simulink model "RoboBoatVU_2014_Athena"  (R2014a)
settings: Solver=FixedStepDiscrete  StartTime=0.0  StopTime=inf  FixedStep=.1  RelTol=1e-3
undefined symbols (not defined in the file): Com1, Com2, Com3, Com4, DiscIntNeverNeededParam, RGB24, standard, strel
libraries: visiontextngfix x25, dspmtrx3 x22, simulink x19, xpcseriallib x12, slrtlib x7, speedgoatlib_IO102 x6, dspstat3 x5, visionstatistics x3, dspindex x2, xpcvideousblib x2, xpcvideoutillib x2, visionmorphops x1
(part 3 of 4)

== system RoboBoatVU_2014_Athena/Main FSM/Return to Start/GPS: Center/Approach ==
  Sensors : Inport
  RGB image : Inport  Port=2
  Enable : EnablePort
  Annotate Task : visiontextngfix/Insert Text  inputType=Obsolete  theText='GPS - Center: Approach - Distance: %f'  getTextLocFrom=Specify via dialog  textLoc=[10 70]  getTextColorFrom=Specify via dialog  textColor=[255 0 0]  getTextIntensityFrom=Specify via dialog  textIntensity=0  getTextOpacityFrom=Specify via dialog  textOpacity=1.0  dummyVar2=0  dummyVar3=0  dummyVar4=0  imagePorts=One multidimensional signal  isInputTransposed=off  fontFace=LucidaSansRegular  dummyVar1=0  blockFontSize=12  antiAliased=on
  Annotate Task2 : visiontextngfix/Insert Text  inputType=Obsolete  theText='Return to Start'  getTextLocFrom=Specify via dialog  textLoc=[1 1]  getTextColorFrom=Specify via dialog  textColor=[0 0 0]  getTextIntensityFrom=Specify via dialog  textIntensity=0  getTextOpacityFrom=Specify via dialog  textOpacity=1.0  dummyVar2=0  dummyVar3=0  dummyVar4=0  imagePorts=One multidimensional signal  isInputTransposed=off  fontFace=LucidaSansRegular  dummyVar1=0  blockFontSize=12  antiAliased=on
  Bus Selector : BusSelector  OutputSignals=Serial In.GPS.latitude,Serial In.GPS.longitude
  Data Store Read : DataStoreRead  DataStoreName=colorGPS  SampleTime=0.1
  Desired Heading and Distance : MATLAB Function  TreatAsAtomicUnit=on
  Output Heirarchy : Subsystem
  Read1 : DataStoreRead  DataStoreName=GPSapproachDist  SampleTime=0.1
  Within Range : MATLAB Function  TreatAsAtomicUnit=on
  Outputs : Outport
  wires:
  Sensors/1 -> Output Heirarchy/4(Sensors), Bus Selector/1  "Sensors"
  Data Store Read/1 -> Desired Heading and Distance/1(DesiredGPS)
  Bus Selector/1 -> Desired Heading and Distance/2(GPSLat)  "<latitude>"
  Bus Selector/2 -> Desired Heading and Distance/3(GPSLong)  "<longitude>"
  Desired Heading and Distance/2(DesiredHeading) -> Output Heirarchy/2(Desired Heading)
  Annotate Task/1 -> Output Heirarchy/3(Annotated Image)
  RGB image/1 -> Annotate Task2/1
  Desired Heading and Distance/1(Distance) -> Annotate Task/2, Within Range/2(Distance)
  Read1/1 -> Within Range/1(GPSApproachDist)
  Within Range/1(Finished) -> Output Heirarchy/1(Finished)  "Task Finished"
  Output Heirarchy/1(Outputs) -> Outputs/1
  Annotate Task2/1 -> Annotate Task/1

== system RoboBoatVU_2014_Athena/Main FSM/Return to Start/GPS: Center/Orient ==
  Sensors : Inport
  RGB image : Inport  Port=2
  Enable : EnablePort
  Annotate Task : visiontextngfix/Insert Text  inputType=Obsolete  theText='GPS - Center: Orient %f'  getTextLocFrom=Specify via dialog  textLoc=[10 70]  getTextColorFrom=Specify via dialog  textColor=[255 0 0]  getTextIntensityFrom=Specify via dialog  textIntensity=0  getTextOpacityFrom=Specify via dialog  textOpacity=1.0  dummyVar2=0  dummyVar3=0  dummyVar4=0  imagePorts=One multidimensional signal  isInputTransposed=off  fontFace=LucidaSansRegular  dummyVar1=0  blockFontSize=12  antiAliased=on
  Annotate Task1 : visiontextngfix/Insert Text  inputType=Obsolete  theText='Current Heading %f'  getTextLocFrom=Specify via dialog  textLoc=[10 40]  getTextColorFrom=Specify via dialog  textColor=[255 0 0]  getTextIntensityFrom=Specify via dialog  textIntensity=0  getTextOpacityFrom=Specify via dialog  textOpacity=1.0  dummyVar2=0  dummyVar3=0  dummyVar4=0  imagePorts=One multidimensional signal  isInputTransposed=off  fontFace=LucidaSansRegular  dummyVar1=0  blockFontSize=12  antiAliased=on
  Annotate Task2 : visiontextngfix/Insert Text  inputType=Obsolete  theText='Return to Start'  getTextLocFrom=Specify via dialog  textLoc=[1 1]  getTextColorFrom=Specify via dialog  textColor=[0 0 0]  getTextIntensityFrom=Specify via dialog  textIntensity=0  getTextOpacityFrom=Specify via dialog  textOpacity=1.0  dummyVar2=0  dummyVar3=0  dummyVar4=0  imagePorts=One multidimensional signal  isInputTransposed=off  fontFace=LucidaSansRegular  dummyVar1=0  blockFontSize=12  antiAliased=on
  Bus Selector : BusSelector  OutputSignals=Serial In.GPS.latitude,Serial In.GPS.longitude,Serial In.Compass.Heading
  Data Store Read : DataStoreRead  DataStoreName=colorGPS  SampleTime=0.1
  Desired Heading : MATLAB Function  TreatAsAtomicUnit=on
  Output Heirarchy1 : Subsystem
  Within Range : MATLAB Function  TreatAsAtomicUnit=on
  Outputs : Outport
  Finished : Outport  Port=2
  wires:
  Sensors/1 -> Output Heirarchy1/3(Sensors), Bus Selector/1  "Sensors"
  Data Store Read/1 -> Desired Heading/1(DesiredGPS)
  Bus Selector/1 -> Desired Heading/2(GPSLat)  "<latitude>"
  Bus Selector/2 -> Desired Heading/3(GPSLong)  "<longitude>"
  Desired Heading/1(DesiredHeading) -> Output Heirarchy1/2(Desired Heading), Annotate Task/2, Within Range/1(DesiredHeading)
  Bus Selector/3 -> Annotate Task1/2, Within Range/2(Compass)  "<Heading>"
  Within Range/1(Finished) -> Finished/1
  RGB image/1 -> Annotate Task2/1
  Output Heirarchy1/1(Outputs) -> Outputs/1
  Annotate Task/1 -> Annotate Task1/1
  Annotate Task1/1 -> Output Heirarchy1/1(Annotated Image)
  Annotate Task2/1 -> Annotate Task/1

== system RoboBoatVU_2014_Athena/Main FSM/Return to Start/GPS: Center/Output Reassign ==
  Outputs in : Inport
  Bus Selector : BusSelector  OutputSignals=Task Finished,Output Signals
  Outputs : Outport
  Finished : Outport  Port=2
  wires:
  Outputs in/1 -> Bus Selector/1
  Bus Selector/1 -> Finished/1  "<Task Finished>"
  Bus Selector/2 -> Outputs/1  "<Output Signals>"

== system RoboBoatVU_2014_Athena/Main FSM/Start Speed Gate/Start Speed Gate - Color/Buoy Decisions ==
  Sensors : Inport
  RGB image : Inport  Port=2
  Red + Green : Inport  Port=3
  Timer : Inport  Port=4
  Annotate Image : Subsystem
  Bus Selector : BusSelector  OutputSignals=Serial In.Compass.Heading
  Bus Selector1 : BusSelector  OutputSignals=Red BBox,Green BBox,Red Centroid,Green Centroid
  Nav Logic : MATLAB Function  TreatAsAtomicUnit=on
  Read : DataStoreRead  DataStoreName=Course
  Annotated Image : Outport
  RPM : Outport  Port=2
  Desired Heading : Outport  Port=3
  wires:
  RGB image/1 -> Annotate Image/1(RGB image)
  Red + Green/1 -> Bus Selector1/1
  Annotate Image/1(Annotated Image) -> Annotated Image/1
  Bus Selector1/1 -> Annotate Image/2(Red BBox), Nav Logic/2(RedBBox)  "<Red BBox>"
  Bus Selector1/2 -> Annotate Image/3(Green BBox), Nav Logic/3(GreenBBox)  "<Green BBox>"
  Bus Selector1/3 -> Nav Logic/4(RedCentroid)  "<Red Centroid>"
  Bus Selector1/4 -> Nav Logic/5(GreenCentroid)  "<Green Centroid>"
  Bus Selector/1 -> Nav Logic/1(Compass)  "<Heading>"
  Sensors/1 -> Bus Selector/1
  Nav Logic/1(RedDist) -> Annotate Image/4(Red Dist)
  Nav Logic/2(GreenDist) -> Annotate Image/5(Green Dist)
  Nav Logic/3(RPM) -> RPM/1
  Nav Logic/4(DesiredHeading) -> Desired Heading/1
  Read/1 -> Nav Logic/6(Course)
  Timer/1 -> Nav Logic/7(Timer)

== system RoboBoatVU_2014_Athena/Main FSM/Start Speed Gate/Start Speed Gate - Color/Output Heirarchy ==
  Sensors : Inport
  Annotated Image : Inport  Port=2
  RPM : Inport  Port=3
  Desired Heading : Inport  Port=4
  Finished : Inport  Port=5
  Bus Creator : BusCreator  Inputs=3
  Bus Creator1 : BusCreator  Inputs=2
  Bus Creator2 : BusCreator  Inputs=3
  Bus Creator3 : BusCreator  Inputs=2
  Bus Creator4 : BusCreator  Inputs=2
  Due Sample Start : Constant  Value=0
  Ready to Read : Constant  Value=0
  Uno Power : Constant  Value=0
  Outputs : Outport
  wires:
  RPM/1 -> Bus Creator/1  "RPM"
  Bus Creator/1 -> Bus Creator1/1  "Control Signals"
  Bus Creator2/1 -> Bus Creator/3  "Arduino Signals"
  Uno Power/1 -> Bus Creator2/2  "Uno Power"
  Desired Heading/1 -> Bus Creator/2  "Desired Heading"
  Bus Creator1/1 -> Bus Creator4/1  "Outputs"
  Annotated Image/1 -> Bus Creator1/2  "Annotated Image"
  Sensors/1 -> Bus Creator4/2  "Sensors"
  Bus Creator4/1 -> Bus Creator3/1  "Output Signals"
  Ready to Read/1 -> Bus Creator2/1  "Ready to Read"
  Due Sample Start/1 -> Bus Creator2/3  "Due Sample Start"
  Finished/1 -> Bus Creator3/2  "Task Finished"
  Bus Creator3/1 -> Outputs/1

== system RoboBoatVU_2014_Athena/Main FSM/Start Speed Gate/Start Speed Gate - Color/Start Speed Gate Detection ==
  RGB : Inport
  Bus Creator : BusCreator
  Green Detection : Subsystem
  Red Detection : Subsystem
  S-Function : S-Function  FunctionName=rgbtohsv_int_sfun  EnableBusSupport=off
  Red + Green : Outport
  wires:
  RGB/1 -> S-Function/1
  S-Function/1 -> Green Detection/1(HSV), Red Detection/1(HSV)
  Red Detection/1(Red Centroid) -> Bus Creator/1  "Red Centroid"
  Red Detection/2(Red BBox) -> Bus Creator/2  "Red BBox"
  Green Detection/1(Green Centroid) -> Bus Creator/3  "Green Centroid"
  Green Detection/2(Green BBox) -> Bus Creator/4  "Green BBox"
  Bus Creator/1 -> Red + Green/1

== matlab function RoboBoatVU_2014_Athena/Parameters/GPS Points/GPS Selector ==
  data: course input; ssGate output; rtnIn input; ssGateA input; colorA input; obstNavStartA input; obstNavEndA input; acouLocA input; dockA input; ssGateB input; colorB input; obstNavStartB input; obstNavEndB input; acouLocB input; dockB input; ssGateT input; colorT input; obstNavStartT input; obstNavEndT input; acouLocT input; dockT input; color output; obstNavStart output; obstNavEnd output; acouLoc output; dock output; rtnOut output
function [ssGate,color,obstNavStart,obstNavEnd,acouLoc,dock,rtnOut] = ...
    GPSselector(course,rtnIn,...
    ssGateA,colorA,obstNavStartA,obstNavEndA,acouLocA,dockA,...
    ssGateB,colorB,obstNavStartB,obstNavEndB,acouLocB,dockB,...
    ssGateT,colorT,obstNavStartT,obstNavEndT,acouLocT,dockT)

%Written by: Anderson Lebbad on July 18, 2013
%Last Edited: Edward Zhu on June
%   Data type mismatch addressed
%   Character conversion redundant

%Selects GPS Points to use based on input Course

%Check value of CourseStr and pass inputs accordingly

switch course
    case uint8('A')
        ssGate = ssGateA;
        color = colorA;
        obstNavStart = obstNavStartA;
        obstNavEnd = obstNavEndA;
        acouLoc = acouLocA;
        dock = dockA;
        rtnOut = rtnIn;
        
    case uint8('B')
        ssGate = ssGateB;
        color = colorB;
        obstNavStart = obstNavStartB;
        obstNavEnd = obstNavEndB;
        acouLoc = acouLocB;
        dock = dockB;
        rtnOut = rtnIn;
        
    otherwise
        ssGate = ssGateT;
        color = colorT;
        obstNavStart = obstNavStartT;
        obstNavEnd = obstNavEndT;
        acouLoc = acouLocT;
        dock = dockT;
        rtnOut = rtnIn;
end

== matlab function RoboBoatVU_2014_Athena/Parameters/Task Selector/Message Composer3 ==
  data: taskStrInit input; taskStrAdj output
function taskStrAdj = composeMessage(taskStrInit)
%Written by Anderson Lebbad on August 9, 2013
%Last Edited: Edward Zhu on June 2, 2014

%This function adjusts the length of a vector to a set value by filling
%the remaining space with 0's. This is necessary for data store objects
%that have a fixed size for the memory allocation, but a variable length
%input.

%Length of message packet
strLength = 8;

%Size of text in message
taskStrLength = size(taskStrInit,1);

%Pad end of text with zeros
taskStrAdj = [taskStrInit' zeros(1,strLength-taskStrLength)];

== matlab function RoboBoatVU_2014_Athena/Parameters/Task Selector/Message Composer6 ==
  data: taskStrInit input; taskStrAdj output
function taskStrAdj = composeMessage(taskStrInit)
%Written by Anderson Lebbad on August 9, 2013
%Last Edited: Edward Zhu on June 2, 2014

%This function adjusts the length of a vector to a set value by filling
%the remaining space with 0's. This is necessary for data store objects
%that have a fixed size for the memory allocation, but a variable length
%input.

%Length of message packet
strLength = 8;

%Size of text in message
taskStrLength = size(taskStrInit,1);

%Pad end of text with zeros
taskStrAdj = [taskStrInit' zeros(1,strLength-taskStrLength)];

== system RoboBoatVU_2014_Athena/Main FSM/Start Speed Gate/Start Speed Gate - LIDAR/Output Heirarchy ==
  Sensors : Inport
  Annotated Image : Inport  Port=2
  RPM : Inport  Port=3
  Desired Heading : Inport  Port=4
  Finished : Inport  Port=5
  Bus Creator : BusCreator  Inputs=3
  Bus Creator1 : BusCreator  Inputs=2
  Bus Creator2 : BusCreator  Inputs=3
  Bus Creator3 : BusCreator  Inputs=2
  Bus Creator4 : BusCreator  Inputs=2
  Due Sample Start : Constant  Value=0
  Ready to Read : Constant  Value=0
  Uno Power : Constant  Value=0
  Outputs : Outport
  wires:
  RPM/1 -> Bus Creator/1  "RPM"
  Bus Creator/1 -> Bus Creator1/1  "Control Signals"
  Bus Creator2/1 -> Bus Creator/3  "Arduino Signals"
  Uno Power/1 -> Bus Creator2/2  "Uno Power"
  Desired Heading/1 -> Bus Creator/2  "Desired Heading"
  Bus Creator1/1 -> Bus Creator4/1  "Outputs"
  Annotated Image/1 -> Bus Creator1/2  "Annotated Image"
  Sensors/1 -> Bus Creator4/2  "Sensors"
  Bus Creator4/1 -> Bus Creator3/1  "Output Signals"
  Ready to Read/1 -> Bus Creator2/1  "Ready to Read"
  Due Sample Start/1 -> Bus Creator2/3  "Due Sample Start"
  Finished/1 -> Bus Creator3/2  "Task Finished"
  Bus Creator3/1 -> Outputs/1

== system RoboBoatVU_2014_Athena/Sensors/Serial In/Decode Compass/Correct Heading Angle Magnetic to True North ==
  Heading Mag : Inport
  Magnetic to True North Conversion : MATLAB Function  TreatAsAtomicUnit=on
  Heading True : Outport
  wires:
  Magnetic to True North Conversion/1(HeadingT) -> Heading True/1  "Heading"
  Heading Mag/1 -> Magnetic to True North Conversion/1(HeadingM)

== system RoboBoatVU_2014_Athena/Sinks/actuators/analog output/Subsystem ==
  Compass Heading : Inport
  Control Signals : Inport  Port=2
  Bus Selector : BusSelector  OutputSignals=RPM,Desired Heading
  Heading Controller : Subsystem
  Propulsion Controller : Subsystem
  Propulsion : Outport
  Steering : Outport  Port=2
  wires:
  Control Signals/1 -> Bus Selector/1
  Bus Selector/1 -> Propulsion Controller/1(RPM)  "<RPM>"
  Propulsion Controller/1(Propulsion) -> Propulsion/1
  Bus Selector/2 -> Heading Controller/1(Heading Desired)  "<Desired Heading>"
  Compass Heading/1 -> Heading Controller/2(Compass Heading)
  Heading Controller/1(Steering) -> Steering/1

== system RoboBoatVU_2014_Athena/Main FSM/Return to Start/GPS: Center/Approach/Output Heirarchy ==
  Finished : Inport
  Desired Heading : Inport  Port=2
  Annotated Image : Inport  Port=3
  Sensors : Inport  Port=4
  Bus Creator : BusCreator  Inputs=3
  Bus Creator1 : BusCreator  Inputs=2
  Bus Creator2 : BusCreator  Inputs=3
  Bus Creator3 : BusCreator  Inputs=2
  Bus Creator4 : BusCreator  Inputs=2
  Due Sample Start : Constant  Value=0
  RPM Desired : Constant  Value=0
  Ready to Read : Constant  Value=0
  Uno Power : Constant  Value=0
  Outputs : Outport
  wires:
  RPM Desired/1 -> Bus Creator/1  "RPM"
  Bus Creator/1 -> Bus Creator1/1  "Control Signals"
  Bus Creator2/1 -> Bus Creator/3  "Arduino Signals"
  Uno Power/1 -> Bus Creator2/2  "Uno Power"
  Desired Heading/1 -> Bus Creator/2  "Desired Heading"
  Bus Creator1/1 -> Bus Creator4/1  "Outputs"
  Annotated Image/1 -> Bus Creator1/2  "Annotated Image"
  Sensors/1 -> Bus Creator4/2  "Sensors"
  Bus Creator4/1 -> Bus Creator3/1  "Output Signals"
  Ready to Read/1 -> Bus Creator2/1  "Ready to Read"
  Due Sample Start/1 -> Bus Creator2/3  "Due Sample Start"
  Bus Creator3/1 -> Outputs/1
  Finished/1 -> Bus Creator3/2  "Task Finished"

== system RoboBoatVU_2014_Athena/Main FSM/Return to Start/GPS: Center/Orient/Output Heirarchy1 ==
  Annotated Image : Inport
  Desired Heading : Inport  Port=2
  Sensors : Inport  Port=3
  Bus Creator : BusCreator  Inputs=3
  Bus Creator1 : BusCreator  Inputs=2
  Bus Creator2 : BusCreator  Inputs=3
  Bus Creator3 : BusCreator  Inputs=2
  Bus Creator4 : BusCreator  Inputs=2
  Due Sample Start : Constant  Value=0
  Finished : Constant  Value=0
  RPM Desired : Constant  Value=0
  Ready to Read : Constant  Value=0
  Uno Power : Constant  Value=0
  Outputs : Outport
  wires:
  RPM Desired/1 -> Bus Creator/1  "RPM"
  Bus Creator/1 -> Bus Creator1/1  "Control Signals"
  Bus Creator2/1 -> Bus Creator/3  "Arduino Signals"
  Uno Power/1 -> Bus Creator2/2  "Uno Power"
  Desired Heading/1 -> Bus Creator/2  "Desired Heading"
  Bus Creator1/1 -> Bus Creator4/1  "Outputs"
  Annotated Image/1 -> Bus Creator1/2  "Annotated Image"
  Sensors/1 -> Bus Creator4/2  "Sensors"
  Bus Creator4/1 -> Bus Creator3/1  "Output Signals"
  Ready to Read/1 -> Bus Creator2/1  "Ready to Read"
  Due Sample Start/1 -> Bus Creator2/3  "Due Sample Start"
  Bus Creator3/1 -> Outputs/1
  Finished/1 -> Bus Creator3/2  "Task Finished"

== system RoboBoatVU_2014_Athena/Main FSM/Start Speed Gate/Start Speed Gate - Color/Buoy Decisions/Annotate Image ==
  RGB image : Inport
  Red BBox : Inport  Port=2
  Green BBox : Inport  Port=3
  Red Dist : Inport  Port=4
  Green Dist : Inport  Port=5
  Annotate Task : visiontextngfix/Insert Text  inputType=Obsolete  theText='Buoy Navigation'  getTextLocFrom=Specify via dialog  textLoc=[10 10]  getTextColorFrom=Specify via dialog  textColor=[0 0 255]  getTextIntensityFrom=Specify via dialog  textIntensity=0  getTextOpacityFrom=Specify via dialog  textOpacity=1.0  dummyVar2=0  dummyVar3=0  dummyVar4=0  imagePorts=One multidimensional signal  isInputTransposed=off  fontFace=LucidaSansRegular  dummyVar1=0  blockFontSize=12  antiAliased=on
  Draw Green BBox : visiontextngfix/Draw Shapes  shape=Rectangles  fill=on  lineWidth=1  fillClrSource=Specify via dialog  display=User-specified value  intensity=200  color=[0 255 0]  opacity=0.6  viewport=Entire image  antialiasing=off  inType=Obsolete  imagePorts=One multidimensional signal  prodOutputMode=Binary point scaling  prodOutputWordLength=32  prodOutputFracLength=14  memoryMode=Specify word length  memoryWordLength=16  memoryFracLength=14  roundingMode=Floor  overflowMode=off
  Draw Red BBox : visiontextngfix/Draw Shapes  shape=Rectangles  fill=on  lineWidth=1  fillClrSource=Specify via dialog  display=User-specified value  intensity=200  color=[255 0 0]  opacity=0.6  viewport=Entire image  antialiasing=off  inType=Obsolete  imagePorts=One multidimensional signal  prodOutputMode=Binary point scaling  prodOutputWordLength=32  prodOutputFracLength=14  memoryMode=Specify word length  memoryWordLength=16  memoryFracLength=14  roundingMode=Floor  overflowMode=off
  Green Distance Display : visiontextngfix/Insert Text  inputType=Obsolete  theText='Green Distance: %f m'  getTextLocFrom=Specify via dialog  textLoc=[10 130]  getTextColorFrom=Specify via dialog  textColor=[0 255 0]  getTextIntensityFrom=Specify via dialog  textIntensity=0  getTextOpacityFrom=Specify via dialog  textOpacity=1.0  dummyVar2=0  dummyVar3=0  dummyVar4=0  imagePorts=One multidimensional signal  isInputTransposed=off  fontFace=LucidaSansRegular  dummyVar1=0  blockFontSize=12  antiAliased=on
  Green integer : DataTypeConversion  OutDataTypeStr=int32
  Red Distance Display : visiontextngfix/Insert Text  inputType=Obsolete  theText='Red Distance: %f m'  getTextLocFrom=Specify via dialog  textLoc=[10 70]  getTextColorFrom=Specify via dialog  textColor=[255 0 0]  getTextIntensityFrom=Specify via dialog  textIntensity=0  getTextOpacityFrom=Specify via dialog  textOpacity=1.0  dummyVar2=0  dummyVar3=0  dummyVar4=0  imagePorts=One multidimensional signal  isInputTransposed=off  fontFace=LucidaSansRegular  dummyVar1=0  blockFontSize=12  antiAliased=on
  Red integer : DataTypeConversion  OutDataTypeStr=int32
  Annotated Image : Outport
  wires:
  RGB image/1 -> Draw Red BBox/1
  Red BBox/1 -> Red integer/1
  Red integer/1 -> Draw Red BBox/2
  Draw Red BBox/1 -> Draw Green BBox/1
  Green BBox/1 -> Green integer/1
  Draw Green BBox/1 -> Annotate Task/1
  Annotate Task/1 -> Red Distance Display/1
  Red Dist/1 -> Red Distance Display/2
  Green Distance Display/1 -> Annotated Image/1
  Red Distance Display/1 -> Green Distance Display/1
  Green Dist/1 -> Green Distance Display/2
  Green integer/1 -> Draw Green BBox/2

== system RoboBoatVU_2014_Athena/Main FSM/Start Speed Gate/Start Speed Gate - Color/Start Speed Gate Detection/Green Detection ==
  HSV : Inport
  Blob Analysis : visionstatistics/Blob Analysis  Tag=vipblks_row_conv  area=on  centroid=on  bBox=on  majorAxis=off  minorAxis=off  angle=off  eccentricity=off  equivDiameterSq=off  extent=on  perimeter=off  maxBlobs=4  warnIfNumBlobsExceeded=on  isCount=off  useMinArea=on  minArea=130  useMaxArea=off  maxArea=6000  excludeBorderBlob=off  outDT=double  isOutVarDim=off  isFill=on  fillValues=-1  conn=8  isLabel=off  outputMode=Binary point scaling  outputWordLength=32  outputFracLength=16  firstCoeffMode=Binary point scaling  firstCoeffWordLength=16  firstCoeffFracLength=14  secondCoeffMode=Binary point scaling  secondCoeffWordLength=32  secondCoeffFracLength=16  accumMode=Binary point scaling  accumWordLength=32  accumFracLength=0  prodOutputMode=Binary point scaling  prodOutputWordLength=32  prodOutputFracLength=16  roundingMode=Floor  overflowMode=off
  Exclusions1 : Subsystem
  Image Reduction : Subsystem
  y-shift : MATLAB Function  Commented=through  TreatAsAtomicUnit=on
  Green Centroid : Outport
  Green BBox : Outport  Port=2
  wires:
  HSV/1 -> Image Reduction/1(HSV)
  Exclusions1/1(Centroid Out) -> y-shift/1(CentroidIn)
  Exclusions1/2(BBox Out) -> y-shift/2(BBoxIn)
  y-shift/1(CentroidOut) -> Green Centroid/1
  y-shift/2(BBoxOut) -> Green BBox/1
  Blob Analysis/2 -> Exclusions1/2(Centroid In)
  Blob Analysis/1 -> Exclusions1/1(Area In)
  Blob Analysis/3 -> Exclusions1/3(BBox In)
  Blob Analysis/4 -> Exclusions1/4(Extent In)
  Image Reduction/1(Green BW) -> Blob Analysis/1

== system RoboBoatVU_2014_Athena/Main FSM/Start Speed Gate/Start Speed Gate - Color/Start Speed Gate Detection/Red Detection ==
  HSV : Inport
  Blob Analysis : visionstatistics/Blob Analysis  Tag=vipblks_row_conv  area=on  centroid=on  bBox=on  majorAxis=off  minorAxis=off  angle=off  eccentricity=off  equivDiameterSq=off  extent=on  perimeter=off  maxBlobs=4  warnIfNumBlobsExceeded=on  isCount=off  useMinArea=on  minArea=130  useMaxArea=off  maxArea=6000  excludeBorderBlob=off  outDT=double  isOutVarDim=off  isFill=on  fillValues=-1  conn=8  isLabel=off  outputMode=Binary point scaling  outputWordLength=32  outputFracLength=16  firstCoeffMode=Binary point scaling  firstCoeffWordLength=16  firstCoeffFracLength=14  secondCoeffMode=Binary point scaling  secondCoeffWordLength=32  secondCoeffFracLength=16  accumMode=Binary point scaling  accumWordLength=32  accumFracLength=0  prodOutputMode=Binary point scaling  prodOutputWordLength=32  prodOutputFracLength=16  roundingMode=Floor  overflowMode=off
  Exclusions : Subsystem
  Image Reduction : Subsystem
  y-shift : MATLAB Function  Commented=through  TreatAsAtomicUnit=on
  Red Centroid : Outport
  Red BBox : Outport  Port=2
  wires:
  HSV/1 -> Image Reduction/1(HSV)
  Exclusions/1(Centroid Out) -> y-shift/1(CentroidIn)
  Exclusions/2(BBox Out) -> y-shift/2(BBoxIn)
  y-shift/2(BBoxOut) -> Red BBox/1
  y-shift/1(CentroidOut) -> Red Centroid/1
  Blob Analysis/4 -> Exclusions/4(Extent In)
  Blob Analysis/2 -> Exclusions/2(Centroid In)
  Blob Analysis/1 -> Exclusions/1(Area In)
  Blob Analysis/3 -> Exclusions/3(BBox In)
  Image Reduction/1(Red BW) -> Blob Analysis/1

== system RoboBoatVU_2014_Athena/Sinks/actuators/analog output/Subsystem/Heading Controller ==
  Heading Desired : Inport
  Compass Heading : Inport  Port=2
  Gain : Gain  Gain=-0.05
  MATLAB Function : MATLAB Function  TreatAsAtomicUnit=on
  Saturation : Saturate  UpperLimit=5  LowerLimit=0
  Sum : Sum  Inputs=++|
  Voltage Nuetral : Constant  Value=2.5
  Steering : Outport
  wires:
  Compass Heading/1 -> MATLAB Function/2(CompassHeading)
  Heading Desired/1 -> MATLAB Function/1(HeadingDesired)
  MATLAB Function/1(steering) -> Gain/1
  Gain/1 -> Sum/2
  Voltage Nuetral/1 -> Sum/1
  Sum/1 -> Saturation/1
  Saturation/1 -> Steering/1

== system RoboBoatVU_2014_Athena/Sinks/actuators/analog output/Subsystem/Propulsion Controller ==
  RPM : Inport
  Saturation : Saturate  UpperLimit=5  LowerLimit=0
  Sum : Sum  Inputs=++|
  Voltage Neutral : Constant  Value=2.5
  Volts / RPM : Gain  Gain=2.5/6000
  Propulsion : Outport
  wires:
  RPM/1 -> Volts / RPM/1
  Volts / RPM/1 -> Sum/2
  Voltage Neutral/1 -> Sum/1
  Sum/1 -> Saturation/1
  Saturation/1 -> Propulsion/1

== system RoboBoatVU_2014_Athena/Main FSM/Start Speed Gate/Start Speed Gate - Color/Start Speed Gate Detection/Green Detection/Exclusions1 ==
  Area In : Inport
  Centroid In : Inport  Port=2
  BBox In : Inport  Port=3
  Extent In : Inport  Port=4
  Closest Blob : Subsystem
  Data Type Conversion : DataTypeConversion  OutDataTypeStr=double
  Extent Exclusion : Subsystem
  Height to Width Exclusion : Subsystem
  Logical Operator : Logic  AllPortsSameDT=off  OutDataTypeStr=boolean
  Variable Selector : dspindex/Variable Selector  NumInputs=3  rowsOrCols=Rows  IdxMode=Variable  Elements=[1 3]  ZerOneIdxMode=One-based  errmode=Clip Index  FillMode=on  FillValues=-1
  Centroid Out : Outport
  BBox Out : Outport  Port=2
  wires:
  Extent In/1 -> Extent Exclusion/1(Extent)
  BBox In/1 -> Data Type Conversion/1
  Height to Width Exclusion/1(Idx) -> Logical Operator/1
  Extent Exclusion/1(Idx) -> Logical Operator/2
  Centroid In/1 -> Variable Selector/2
  Closest Blob/1(Centroid Out) -> Centroid Out/1
  Closest Blob/2(BBox Out) -> BBox Out/1
  Data Type Conversion/1 -> Variable Selector/3, Height to Width Exclusion/1(BBox)
  Logical Operator/1 -> Variable Selector/4
  Variable Selector/3 -> Closest Blob/3(BBox In)
  Variable Selector/2 -> Closest Blob/2(Centroid In)
  Variable Selector/1 -> Closest Blob/1(Area In)
  Area In/1 -> Variable Selector/1

== system RoboBoatVU_2014_Athena/Main FSM/Start Speed Gate/Start Speed Gate - Color/Start Speed Gate Detection/Green Detection/Image Reduction ==
  HSV : Inport
  Cut Out Sky : dspmtrx3/Submatrix  RowSpan=Range of rows  RowStartMode=First  RowStartIndex=1  RowEndMode=Index  RowEndIndex=280  ColSpan=Range of columns  ColStartMode=First  ColStartIndex=1  ColEndMode=Last  ColEndIndex=1
  Cut Out Sky1 : dspmtrx3/Submatrix  RowSpan=Range of rows  RowStartMode=First  RowStartIndex=1  RowEndMode=Index  RowEndIndex=280  ColSpan=Range of columns  ColStartMode=First  ColStartIndex=1  ColEndMode=Last  ColEndIndex=1
  H : Selector  NumberOfDimensions=3  InputPortWidth=3  IndexOptions=Select all,Select all,Index vector (dialog)  Indices=[1 3],1,1  OutputSizes=1,1,1
  Logical Operator : Logic  AllPortsSameDT=off  OutDataTypeStr=boolean
  Logical Operator1 : Logic  AllPortsSameDT=off  OutDataTypeStr=boolean
  Logical Operator2 : Logic  AllPortsSameDT=off  OutDataTypeStr=boolean
  Upper limit : simulink/Logic and Bit Operations/Compare To Constant  relop=<=  const=110  OutDataTypeStr=boolean
  Upper limit1 : simulink/Logic and Bit Operations/Compare To Constant  relop=>=  const=90  OutDataTypeStr=boolean
  Upper limit2 : simulink/Logic and Bit Operations/Compare To Constant  relop=>=  const=60  OutDataTypeStr=boolean
  Upper limit3 : simulink/Logic and Bit Operations/Compare To Constant  relop=<=  const=160  OutDataTypeStr=boolean
  V : Selector  NumberOfDimensions=3  InputPortWidth=3  IndexOptions=Select all,Select all,Index vector (dialog)  Indices=[1 3],1,3  OutputSizes=1,1,1
  Green BW : Outport
  wires:
  H/1 -> Cut Out Sky/1
  HSV/1 -> V/1, H/1
  Cut Out Sky/1 -> Upper limit1/1, Upper limit/1
  Upper limit1/1 -> Logical Operator/2
  Upper limit/1 -> Logical Operator/1
  V/1 -> Cut Out Sky1/1
  Cut Out Sky1/1 -> Upper limit3/1, Upper limit2/1
  Logical Operator/1 -> Logical Operator1/1
  Logical Operator1/1 -> Green BW/1
  Upper limit2/1 -> Logical Operator2/1
  Upper limit3/1 -> Logical Operator2/2
  Logical Operator2/1 -> Logical Operator1/2

== system RoboBoatVU_2014_Athena/Main FSM/Start Speed Gate/Start Speed Gate - Color/Start Speed Gate Detection/Red Detection/Exclusions ==
  Area In : Inport
  Centroid In : Inport  Port=2
  BBox In : Inport  Port=3
  Extent In : Inport  Port=4
  Closest Blob : Subsystem
  Data Type Conversion : DataTypeConversion  OutDataTypeStr=double
  Extent Exclusion : Subsystem
  Height to Width Exclusion : Subsystem
  Logical Operator : Logic  AllPortsSameDT=off  OutDataTypeStr=boolean
  Variable Selector : dspindex/Variable Selector  NumInputs=3  rowsOrCols=Rows  IdxMode=Variable  Elements=[1 3]  ZerOneIdxMode=One-based  errmode=Clip Index  FillMode=on  FillValues=-1
  Centroid Out : Outport
  BBox Out : Outport  Port=2
  wires:
  Extent In/1 -> Extent Exclusion/1(Extent)
  BBox In/1 -> Data Type Conversion/1
  Height to Width Exclusion/1(Idx) -> Logical Operator/1
  Extent Exclusion/1(Idx) -> Logical Operator/2
  Logical Operator/1 -> Variable Selector/4
  Centroid In/1 -> Variable Selector/2
  Variable Selector/2 -> Closest Blob/2(Centroid In)
  Variable Selector/3 -> Closest Blob/3(BBox In)
  Closest Blob/1(Centroid Out) -> Centroid Out/1
  Closest Blob/2(BBox Out) -> BBox Out/1
  Data Type Conversion/1 -> Variable Selector/3, Height to Width Exclusion/1(BBox)
  Area In/1 -> Variable Selector/1
  Variable Selector/1 -> Closest Blob/1(Area In)

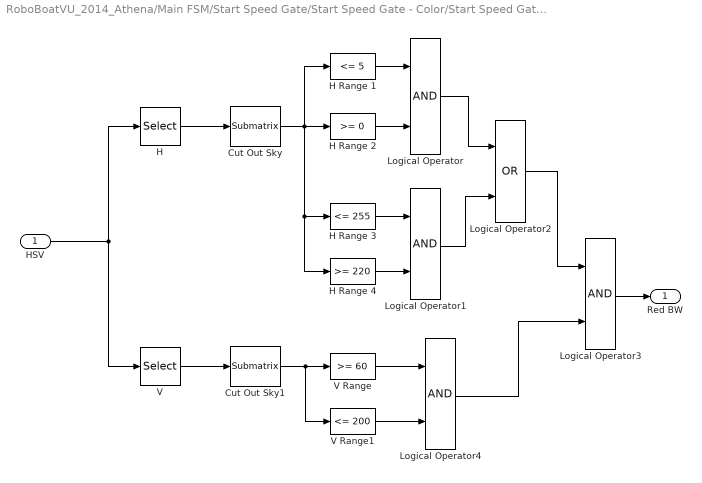
== system RoboBoatVU_2014_Athena/Main FSM/Start Speed Gate/Start Speed Gate - Color/Start Speed Gate Detection/Red Detection/Image Reduction ==
  HSV : Inport
  Cut Out Sky : dspmtrx3/Submatrix  RowSpan=Range of rows  RowStartMode=First  RowStartIndex=1  RowEndMode=Index  RowEndIndex=280  ColSpan=Range of columns  ColStartMode=First  ColStartIndex=1  ColEndMode=Last  ColEndIndex=1
  Cut Out Sky1 : dspmtrx3/Submatrix  RowSpan=Range of rows  RowStartMode=First  RowStartIndex=1  RowEndMode=Index  RowEndIndex=280  ColSpan=Range of columns  ColStartMode=First  ColStartIndex=1  ColEndMode=Last  ColEndIndex=1
  H : Selector  NumberOfDimensions=3  InputPortWidth=3  IndexOptions=Select all,Select all,Index vector (dialog)  Indices=[1 3],1,1  OutputSizes=1,1,1
  H Range 1 : simulink/Logic and Bit Operations/Compare To Constant  relop=<=  const=5  OutDataTypeStr=boolean
  H Range 2 : simulink/Logic and Bit Operations/Compare To Constant  relop=>=  const=0  OutDataTypeStr=boolean
  H Range 3 : simulink/Logic and Bit Operations/Compare To Constant  relop=<=  const=255  OutDataTypeStr=boolean
  H Range 4 : simulink/Logic and Bit Operations/Compare To Constant  relop=>=  const=220  OutDataTypeStr=boolean
  Logical Operator{,1,3..4} (4 alike) : Logic  AllPortsSameDT=off  OutDataTypeStr=boolean
  Logical Operator2 : Logic  Operator=OR  AllPortsSameDT=off  OutDataTypeStr=boolean
  V : Selector  NumberOfDimensions=3  InputPortWidth=3  IndexOptions=Select all,Select all,Index vector (dialog)  Indices=[1 3],1,3  OutputSizes=1,1,1
  V Range : simulink/Logic and Bit Operations/Compare To Constant  relop=>=  const=60  OutDataTypeStr=boolean
  V Range1 : simulink/Logic and Bit Operations/Compare To Constant  relop=<=  const=200  OutDataTypeStr=boolean
  Red BW : Outport
  wires:
  HSV/1 -> H/1, V/1
  H/1 -> Cut Out Sky/1
  Cut Out Sky/1 -> H Range 4/1, H Range 3/1, H Range 2/1, H Range 1/1
  V/1 -> Cut Out Sky1/1
  H Range 1/1 -> Logical Operator/1
  H Range 2/1 -> Logical Operator/2
  H Range 3/1 -> Logical Operator1/1
  H Range 4/1 -> Logical Operator1/2
  Logical Operator/1 -> Logical Operator2/1
  Logical Operator1/1 -> Logical Operator2/2
  Cut Out Sky1/1 -> V Range1/1, V Range/1
  Logical Operator2/1 -> Logical Operator3/1
  Logical Operator3/1 -> Red BW/1
  V Range/1 -> Logical Operator4/1
  V Range1/1 -> Logical Operator4/2
  Logical Operator4/1 -> Logical Operator3/2

== system RoboBoatVU_2014_Athena/Main FSM/Start Speed Gate/Start Speed Gate - Color/Start Speed Gate Detection/Green Detection/Exclusions1/Closest Blob ==
  note: Sorts the list of viable buoys based on the Y location of the bounding box, those
      | with higher values are lower on the screen. The lower the blob is on the screen,
      | the closer it is to the boat, since all the buoys are floating on the surface of the water.
      | The submatrix then selects the centroid and bbox of the blob with the highest
      | Y value and passes it as the closest blob.
  Area In : Inport
  Centroid In : Inport  Port=2
  BBox In : Inport  Port=3
  BBox Select : dspmtrx3/Submatrix  RowSpan=One row  RowStartMode=First  RowStartIndex=1  RowEndMode=Last  RowEndIndex=1  ColSpan=Range of columns  ColStartMode=Index  ColStartIndex=3  ColEndMode=Last  ColEndIndex=1
  Centroid Select : dspmtrx3/Submatrix  RowSpan=One row  RowStartMode=First  RowStartIndex=1  RowEndMode=Last  RowEndIndex=1  ColSpan=Range of columns  ColStartMode=First  ColStartIndex=2  ColEndMode=Index  ColEndIndex=2
  Matrix Concatenate : Concatenate  Mode=Multidimensional array  ConcatenateDimension=2
  Permute Matrix : dspmtrx3/Permute Matrix  mode=Rows  ZeroOneIdxMode=One-based  errmode=Clip index  checkDims=off
  Sort : dspstat3/Sort  otype=Index  dir=Descending  sortAlg=Quick sort  accumDataTypeStr=Inherit: Same as product output  accumLastDataTypeStr=Inherit: Same as product output  roundingMode=Floor  overflowMode=off
  Centroid Out : Outport
  BBox Out : Outport  Port=2
  wires:
  Centroid In/1 -> Matrix Concatenate/1
  BBox In/1 -> Matrix Concatenate/2
  Matrix Concatenate/1 -> Permute Matrix/1
  Sort/1 -> Permute Matrix/2
  Permute Matrix/1 -> BBox Select/1, Centroid Select/1
  BBox Select/1 -> BBox Out/1
  Centroid Select/1 -> Centroid Out/1
  Area In/1 -> Sort/1

== system RoboBoatVU_2014_Athena/Main FSM/Start Speed Gate/Start Speed Gate - Color/Start Speed Gate Detection/Green Detection/Exclusions1/Extent Exclusion ==
  note: Pixels Occpied by blob within bounding box should
      | be within a certain ratio for buoy
  Extent : Inport
  Logical Operator : Logic  AllPortsSameDT=off  OutDataTypeStr=boolean
  Lower limit : simulink/Logic and Bit Operations/Compare To Constant  relop=>=  const=0.4  OutDataTypeStr=boolean
  Upper limit : simulink/Logic and Bit Operations/Compare To Constant  relop=<=  const=0.9  OutDataTypeStr=boolean
  Idx : Outport
  wires:
  Extent/1 -> Lower limit/1, Upper limit/1
  Upper limit/1 -> Logical Operator/1
  Lower limit/1 -> Logical Operator/2
  Logical Operator/1 -> Idx/1

== system RoboBoatVU_2014_Athena/Main FSM/Start Speed Gate/Start Speed Gate - Color/Start Speed Gate Detection/Green Detection/Exclusions1/Height to Width Exclusion ==
  note: Buoys can be percieved significantly taller than they are wide
      | due to relfections in the water, but should not be percieved
      | much wider than they are tall - even in oversaturated lighting
      | conditions (which generally cuts off some height, but doesn't
      | effect width)
  BBox : Inport
  Divide : Product  Inputs=*/
  Height : dspmtrx3/Submatrix  RowSpan=All rows  RowStartMode=First  RowStartIndex=1  RowEndMode=Last  RowEndIndex=1  ColSpan=One column  ColStartMode=Index  ColStartIndex=4  ColEndMode=Last  ColEndIndex=1
  Logical Operator : Logic  AllPortsSameDT=off  OutDataTypeStr=boolean
  Width : dspmtrx3/Submatrix  RowSpan=All rows  RowStartMode=First  RowStartIndex=1  RowEndMode=Last  RowEndIndex=1  ColSpan=One column  ColStartMode=Index  ColStartIndex=3  ColEndMode=Last  ColEndIndex=1
  ratio max : simulink/Logic and Bit Operations/Compare To Constant  relop=<=  const=5  OutDataTypeStr=boolean
  ratio min : simulink/Logic and Bit Operations/Compare To Constant  relop=>=  const=1.5  OutDataTypeStr=boolean
  Idx : Outport
  wires:
  BBox/1 -> Height/1, Width/1
  Height/1 -> Divide/1
  Width/1 -> Divide/2
  Divide/1 -> ratio min/1, ratio max/1
  ratio max/1 -> Logical Operator/1
  ratio min/1 -> Logical Operator/2
  Logical Operator/1 -> Idx/1

== system RoboBoatVU_2014_Athena/Main FSM/Start Speed Gate/Start Speed Gate - Color/Start Speed Gate Detection/Red Detection/Exclusions/Closest Blob ==
  note: Sorts the list of viable buoys based on the Y location of the bounding box, those
      | with higher values are lower on the screen. The lower the blob is on the screen,
      | the closer it is to the boat, since all the buoys are floating on the surface of the water.
      | The submatrix then selects the centroid and bbox of the blob with the highest
      | Y value and passes it as the closest blob.
  Area In : Inport
  Centroid In : Inport  Port=2
  BBox In : Inport  Port=3
  BBox Select : dspmtrx3/Submatrix  RowSpan=One row  RowStartMode=First  RowStartIndex=1  RowEndMode=Last  RowEndIndex=1  ColSpan=Range of columns  ColStartMode=Index  ColStartIndex=3  ColEndMode=Last  ColEndIndex=1
  Centroid Select : dspmtrx3/Submatrix  RowSpan=One row  RowStartMode=First  RowStartIndex=1  RowEndMode=Last  RowEndIndex=1  ColSpan=Range of columns  ColStartMode=First  ColStartIndex=2  ColEndMode=Index  ColEndIndex=2
  Matrix Concatenate : Concatenate  Mode=Multidimensional array  ConcatenateDimension=2
  Permute Matrix : dspmtrx3/Permute Matrix  mode=Rows  ZeroOneIdxMode=One-based  errmode=Clip index  checkDims=off
  Sort : dspstat3/Sort  otype=Index  dir=Descending  sortAlg=Quick sort  accumDataTypeStr=Inherit: Same as product output  accumLastDataTypeStr=Inherit: Same as product output  roundingMode=Floor  overflowMode=off
  Centroid Out : Outport
  BBox Out : Outport  Port=2
  wires:
  Centroid In/1 -> Matrix Concatenate/1
  BBox In/1 -> Matrix Concatenate/2
  Area In/1 -> Sort/1
  Matrix Concatenate/1 -> Permute Matrix/1
  Sort/1 -> Permute Matrix/2
  Permute Matrix/1 -> BBox Select/1, Centroid Select/1
  BBox Select/1 -> BBox Out/1
  Centroid Select/1 -> Centroid Out/1

== system RoboBoatVU_2014_Athena/Main FSM/Start Speed Gate/Start Speed Gate - Color/Start Speed Gate Detection/Red Detection/Exclusions/Extent Exclusion ==
  note: Pixels Occpied by blob within bounding box should
      | be within a certain ratio for buoy
  Extent : Inport
  Logical Operator : Logic  AllPortsSameDT=off  OutDataTypeStr=boolean
  Lower limit : simulink/Logic and Bit Operations/Compare To Constant  relop=>=  const=0.35  OutDataTypeStr=boolean
  Upper limit : simulink/Logic and Bit Operations/Compare To Constant  relop=<=  const=0.9  OutDataTypeStr=boolean
  Idx : Outport
  wires:
  Upper limit/1 -> Logical Operator/1
  Lower limit/1 -> Logical Operator/2
  Logical Operator/1 -> Idx/1
  Extent/1 -> Lower limit/1, Upper limit/1

== system RoboBoatVU_2014_Athena/Main FSM/Start Speed Gate/Start Speed Gate - Color/Start Speed Gate Detection/Red Detection/Exclusions/Height to Width Exclusion ==
  note: Buoys can be percieved significantly taller than they are wide
      | due to relfections in the water, but should not be percieved
      | much wider than they are tall - even in oversaturated lighting
      | conditions (which generally cuts off some height, but doesn't
      | effect width)
  BBox : Inport
  Divide : Product  Inputs=*/
  Height : dspmtrx3/Submatrix  RowSpan=All rows  RowStartMode=First  RowStartIndex=1  RowEndMode=Last  RowEndIndex=1  ColSpan=One column  ColStartMode=Index  ColStartIndex=4  ColEndMode=Last  ColEndIndex=1
  Logical Operator : Logic  AllPortsSameDT=off  OutDataTypeStr=boolean
  Width : dspmtrx3/Submatrix  RowSpan=All rows  RowStartMode=First  RowStartIndex=1  RowEndMode=Last  RowEndIndex=1  ColSpan=One column  ColStartMode=Index  ColStartIndex=3  ColEndMode=Last  ColEndIndex=1
  ratio max : simulink/Logic and Bit Operations/Compare To Constant  relop=<=  const=5  OutDataTypeStr=boolean
  ratio min : simulink/Logic and Bit Operations/Compare To Constant  relop=>=  const=1.5  OutDataTypeStr=boolean
  Idx : Outport
  wires:
  BBox/1 -> Height/1, Width/1
  Height/1 -> Divide/1
  Width/1 -> Divide/2
  Divide/1 -> ratio min/1, ratio max/1
  ratio max/1 -> Logical Operator/1
  ratio min/1 -> Logical Operator/2
  Logical Operator/1 -> Idx/1

== matlab function RoboBoatVU_2014_Athena/Main FSM/Main Enabler ==
  data: taskSelector output; initEn output; colorSeqEn output; ssGateEn output; obstNavEn output; acouLocEn output; dockEn output; rtnEn output; RCEn output; mainTask input; RCHold input; initFin input; colorSeqFin input; ssGateFin input; obstNavFin input; acouLocFin input; dockFin input; rtnFin input; termEn output
function [taskSelector,initEn,colorSeqEn,ssGateEn,obstNavEn,...
    acouLocEn,dockEn,rtnEn,RCEn,termEn] = taskEnabler(mainTask,RCHold,initFin,...
    colorSeqFin,ssGateFin,obstNavFin,acouLocFin,dockFin,rtnFin)
%Written by Anderson Lebbad on July 19, 2013
%Last Edited: Edward Zhu on June 2, 2014
%   Substring search for task was written in
%   Case switches were redundant, combined with first set of if statements

%Changes the value of MainMode and the enablers for the tasks within the 
%Main FSM.

% Initialize enable signals
RCEn = 0;
initEn = 0;
colorSeqEn = 0; 
ssGateEn = 0;
obstNavEn = 0;
acouLocEn = 0;
dockEn = 0;
rtnEn = 0;
termEn = 0;

% Convert main task indicator to a string
mainTaskStr = char(mainTask');

% Adjust finished states based on user task selection
if ~isempty(strfind(mainTaskStr,'Color'))
    initFin = 1;
elseif ~isempty(strfind(mainTaskStr,'SSGate'))
    initFin = 1;
    colorSeqFin = 1;
elseif ~isempty(strfind(mainTaskStr,'Obstacle'))
    initFin = 1;
    colorSeqFin = 1;
    ssGateFin = 1;
elseif ~isempty(strfind(mainTaskStr,'Acoustic'))
    initFin = 1;
    colorSeqFin = 1;
    ssGateFin = 1;
    obstNavFin = 1;
elseif ~isempty(strfind(mainTaskStr,'Dock'))
    initFin = 1;
    colorSeqFin = 1;
    ssGateFin = 1;
    obstNavFin = 1;
    acouLocFin = 1;
elseif ~isempty(strfind(mainTaskStr,'Return'))
    initFin = 1;
    colorSeqFin = 1;
    ssGateFin = 1;
    obstNavFin = 1;
    acouLocFin = 1;
    dockFin = 1;
end

% Set enable signals based on state completion
if initFin == 0
    initEn = 1;
    taskSelector = 1;
elseif RCHold == 0
    RCEn = 1;
    taskSelector = 8;
elseif colorSeqFin == 0
    colorSeqEn = 1;
    taskSelector = 2;
elseif ssGateFin == 0
    ssGateEn = 1;
    taskSelector = 3;
elseif obstNavFin == 0
    obstNavEn = 1;
    taskSelector = 4;
elseif acouLocFin == 0
    acouLocEn = 1;
    taskSelector = 5;
elseif dockFin == 0
    dockEn = 1;
    taskSelector = 6;
elseif rtnFin == 0
    rtnEn = 1;
    taskSelector = 7;
else
    termEn = 1;
    taskSelector = 9;
end

== matlab function RoboBoatVU_2014_Athena/Main FSM/Start Speed Gate/Start Speed Gate - Color/Start Speed Gate Detection/Green Detection/y-shift ==
  data: CentroidIn input; CentroidOut output; BBoxIn input; BBoxOut output
function [CentroidOut, BBoxOut] = yShift(CentroidIn, BBoxIn)

%Written by Anderson Lebbad on July 24, 2013
%Last Edited: Anderson Lebbad on August 4, 2013
%   Renamed the function to match other instances

%This function compensates for the amount of the image that was cut out
%when the sky was removed by the image reduction subsystem

CentroidOut = [CentroidIn(1), CentroidIn(2)+175];
BBoxOut = [BBoxIn(1), BBoxIn(2)+175, BBoxIn(3:4)];

== matlab function RoboBoatVU_2014_Athena/Sinks/actuators/analog output/Subsystem/Heading Controller/MATLAB Function ==
  data: HeadingDesired input; steering output; CompassHeading input
function steering = CalcSteering(HeadingDesired, CompassHeading)

%Written by Anderson Lebbad on July 19, 2013
%Last Edited: Anderson Lebbad on August 14, 2013
%   Simplified using mod division

%Calculates the difference between the desired and current heading to be
%used for steering


%difference is calculated in the range of -180 to 180
steering = mod(HeadingDesired - CompassHeading, 360);
if steering > 180
    steering = steering - 360;
end

== matlab function RoboBoatVU_2014_Athena/Main FSM/Start Speed Gate/Start Speed Gate - Color/Start Speed Gate Detection/Red Detection/y-shift ==
  data: CentroidIn input; CentroidOut output; BBoxIn input; BBoxOut output
function [CentroidOut, BBoxOut] = yShift(CentroidIn, BBoxIn)

%Written by Anderson Lebbad on July 24, 2013
%Last Edited: Anderson Lebbad on August 4, 2013
%   Renamed the function to match other instances

%This function compensates for the amount of the image that was cut out
%when the sky was removed by the image reduction subsystem

CentroidOut = [CentroidIn(1), CentroidIn(2)+175];
BBoxOut = [BBoxIn(1), BBoxIn(2)+175, BBoxIn(3:4)];

== matlab function RoboBoatVU_2014_Athena/Main FSM/Docking/Detection/Detection ==
  data: cruciform input; circle input; triangle input; whitePixCount input; threshold input; V_mask input; bbox_in input; bbox_out output; label input; rtnRatioDiff output
function [bbox_out,rtnRatioDiff]= detection(cruciform,circle,triangle,...
    whitePixCount,threshold,V_mask,bbox_in,label)

% Written by Edward Zhu on 5/14/14

% Inputs
% tempID:       Number corresponding to one of the templates (cruciform: 1,
%               circle: 2, triangle: 3)
% cruciform:    19*19 template of cruciform
% circle:       19*19 template of circle
% triangle:     19*19 template of triangle
% whitePixCount:Number of white pixels in each of the templates
% V_mask:       V channel binary mask
% bbox_in:      Bounding boxes as found by blob analysis
% label:        Label matrix as found by blob analysis

% Outputs
% bbox_out:     Bounding box of matched symbol
% symFound:     Status of matching (found: 1, not found: 0)

% Define frame and template size
templates = zeros(19,19,3);
templates(:,:,1) = cruciform;
templates(:,:,2) = circle;
templates(:,:,3) = triangle;

imgRows = size(label,1);
imgCols = size(label,2);
tempRows = size(templates,1);
tempCols = size(templates,2);
numBBox = size(bbox_in,1);

% Initialize scaled image and output bbox matrices
V_scaled = zeros(tempRows,tempCols);
bbox_out = uint32(zeros(numBBox,4));
rtnRatioDiff = ones(numBBox,1);

bestRatioDiff = single(1);

for i = 1:numBBox
    shapeDiff = abs(1-bbox_in(i,3)/bbox_in(i,4));
    if bbox_in(i,3) >= tempCols && bbox_in(i,4) >= tempRows && shapeDiff < 0.5
        % Set up arrays for the start and end rows and columns for bbox
        % matching
        
        similarity = zeros(1,3);
        ratioDiff = zeros(1,3);
        
        rowStep = floor(bbox_in(i,4) / tempRows);
        colStep = floor(bbox_in(i,3) / tempCols);
        
        startRowList = zeros(1,3);
        startRowList(2) = bbox_in(i,2);
        startRowList(1) = max(1, startRowList(2) - rowStep);
        startRowList(3) = min(imgRows, startRowList(2) + rowStep);
        
        endRowList = zeros(1,3);
        endRowList(2) = bbox_in(i,2) + bbox_in(i,4);
        endRowList(1) = max(1, endRowList(2) - rowStep);
        endRowList(3) = min(imgRows, endRowList(2) + rowStep);
        
        startColList = zeros(1,3);
        startColList(2) = bbox_in(i,1);
        startColList(1) = max(1, startColList(2) - colStep);
        startColList(3) = min(imgCols, startColList(2) + colStep);
        
        endColList = zeros(1,3);
        endColList(2) = bbox_in(i,1) + bbox_in(i,3);
        endColList(1) = max(1, endColList(2) - colStep);
        endColList(3) = min(imgCols, endColList(2) + colStep);
        
        % Scale down image in bbox to size of template (18*18 px)
        for startRow = startRowList
            for endRow = endRowList
                rowScaleStep = floor((endRow - startRow) / tempRows);
                
                for startCol = startColList
                    for endCol = endColList
                        colScaleStep = floor((endCol - startCol) / tempCols);
                        
                        captureRow = startRow;
                        for row = 1:tempRows
                            captureCol = startCol;
                            for col = 1:tempCols
                                V_scaled(row,col) = V_mask(captureRow,captureCol);
                                for tempID = 1:3
                                    similarity(tempID) = similarity(tempID) + templates(row,col,tempID) * (V_mask(captureRow,captureCol)*(-1) + 1);
                                end
                                captureCol = captureCol + colScaleStep;                        
                            end
                            captureRow = captureRow + rowScaleStep;
                        end                  
                        
                        for tempID = 1:3   
                            ratioDiff(tempID) = abs(1 - single(similarity(tempID)) / single(whitePixCount(tempID))); 
                        end
                        
                        if min(ratioDiff) < bestRatioDiff
                            bestRatioDiff = single(min(ratioDiff));
                        end
                    end
                end
            end
        end
        
        % Output valid bounding boxes
        if bestRatioDiff < threshold
            bbox_out(i,:) = bbox_in(i,:);
            rtnRatioDiff(i) = bestRatioDiff;
        end
    end
end

== matlab function RoboBoatVU_2014_Athena/Main FSM/Docking/MATLAB Function ==
  data: xRec input; xDet input; bayNumber output
function bayNumber = bayPosition(xRec,xDet)

symxpos = xRec(1);

diff1 = xDet(1) - symxpos;
diff2 = xDet(2) - symxpos;
diff3 = xDet(3) - symxpos;

if diff1 == 0
    bayNumber = uint8(1);
elseif diff2 == 0
    bayNumber = uint8(2);
elseif diff3 == 0
    bayNumber = uint8(3);
else
    bayNumber = uint8(0);
end
